simulink model "Copy_of_bird"  (R2022a)
settings: Solver=VariableStepAuto  StartTime=0.0  StopTime=250.0  RelTol=1e-3
settings Model: PacingRate=1000  Creator=violet_in_summer  LastModifiedBy=violet_in_summer

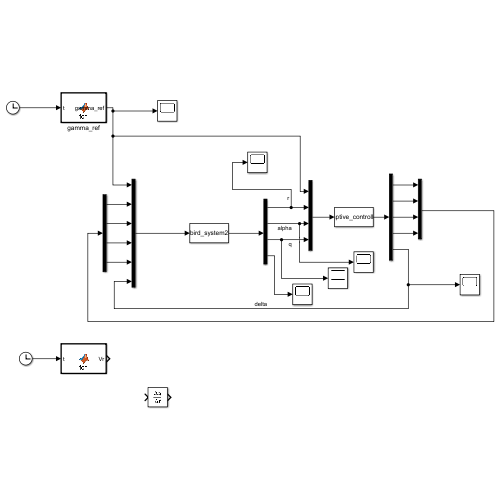
[thumbnail: Simulink's stored preview of the top-level diagram]
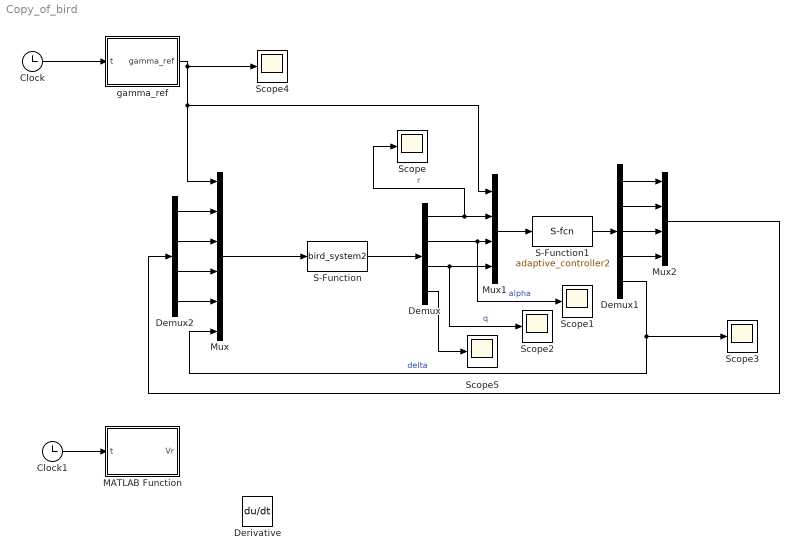
== system Copy_of_bird ==
  Clock : Clock
  Clock1 : Clock
  Demux : Demux
  Demux1 : Demux  Outputs=5
  Demux2 : Demux
  Derivative : Derivative
  MATLAB Function : MATLAB Function  TreatAsAtomicUnit=on
  Mux : Mux  Inputs=6
  Mux1 : Mux
  Mux2 : Mux
  S-Function : S-Function  FunctionName=bird_system2  Parameters=para  SFunctionDeploymentMode=off  EnableBusSupport=off
  S-Function1 : S-Function  FunctionName=adaptive_controller2  Parameters=para  SFunctionDeploymentMode=off  EnableBusSupport=off
  Scope{,1..5} (6 alike) : Scope
  gamma_ref : MATLAB Function  TreatAsAtomicUnit=on
  wires:
  Mux/1 -> S-Function/1
  S-Function/1 -> Demux/1
  Mux1/1 -> S-Function1/1
  S-Function1/1 -> Demux1/1
  Clock/1 -> gamma_ref/1(t)
  gamma_ref/1(gamma_ref) -> Scope4/1, Mux1/1, Mux/1
  Demux1/1 -> Mux2/1
  Demux1/2 -> Mux2/2
  Demux1/3 -> Mux2/3
  Demux1/4 -> Mux2/4
  Demux1/5 -> Scope3/1, Mux/6  "delta"
  Demux/1 -> Scope/1, Mux1/2  "r"
  Demux/2 -> Scope1/1, Mux1/3  "alpha"
  Demux/3 -> Mux1/4, Scope2/1  "q"
  Mux2/1 -> Demux2/1
  Demux2/1 -> Mux/2
  Demux2/2 -> Mux/3
  Demux2/3 -> Mux/4
  Demux2/4 -> Mux/5
  Demux/4 -> Scope5/1
  Clock1/1 -> MATLAB Function/1(t)

== matlab function Copy_of_bird/gamma_ref ==
  data: t input; gamma_ref output
function gamma_ref = fcn(t)
if (t>=0) && (t<20)
    gamma_ref = 0;
elseif (t>=20) && (t<50)
    gamma_ref = 10;
elseif (t>=50) && (t<80)
    gamma_ref = 5;
elseif (t>=80) && (t<120)
    gamma_ref = -3;
elseif (t>=120) && (t<160)
    gamma_ref = 4;
else
    gamma_ref = 0;
end

== matlab function Copy_of_bird/MATLAB Function ==
  data: t input; Vr output
function Vr = fcn(t)
if (t>=0) && (t<80)
    Vr = 80;
elseif (t>=80) && (t<150)
    Vr = (105-80)/(150-80) * t;
elseif (t>=150) && (t<170)
    Vr = 105;
elseif (t>=170) && (t<200)
    Vr = (72-105)/(200-170) * t;
else
    Vr = 72;
end
